simulink model "EXP7_Part2"  (R2018a)
settings: Solver=VariableStepAuto  StartTime=0.0  StopTime=0.2  RelTol=1e-3
undefined symbols (not defined in the file): DiscIntNeverNeededParam
libraries: dsparch4 x1, commsynccomp2 x1, dspsrcs4 x1
settings Model: Creator=user  LastModifiedBy=shohan

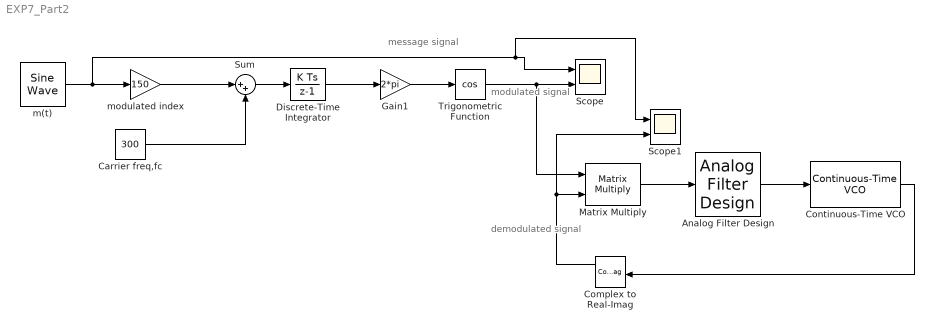
== system EXP7_Part2 ==
  note: modulated signal
  note: message signal
  note: demodulated
      | signal
  Analog Filter Design : dsparch4/Analog Filter Design  method=Butterworth  filttype=Lowpass  N=10  Wlo=2*pi*5  Whi=80  Rp=2  Rs=40
  Carrier freq,fc : Constant  Value=300
  Complex to Real-Imag : ComplexToRealImag
  Continuous-Time VCO : commsynccomp2/Continuous-Time VCO  Ac=1  Fc=10  Kc=50  Ph=0
      settings: SourceProductName=Communications System Toolbox  SourceProductBaseCode=CM
  Discrete-Time Integrator : DiscreteIntegrator  SampleTime=1/98000  ICPrevOutput=DiscIntNeverNeededParam  ICPrevScaledInput=DiscIntNeverNeededParam
  Gain1 : Gain  Gain=2*pi
  Matrix Multiply : Product  Multiplication=Matrix(*)
  Scope : Scope  NumInputPorts=2
  Scope1 : Scope  NumInputPorts=2
  Sum : Sum  Inputs=|++
  Trigonometric Function : Trigonometry  Operator=cos
  m(t) : dspsrcs4/Sine Wave  Amplitude=2  Frequency=10  Phase=pi/3  SampleMode=Discrete  OutComplex=Real  CompMethod=Trigonometric fcn  TableSize=Speed  SampleTime=1/98000  SamplesPerFrame=1  ResetState=Restart at time zero  OutputFrames=off  dataType=double  wordLen=16  udDataType=sfix(16)  fracBitsMode=Best precision  numFracBits=15  OutDataTypeStr=double  LastOutDataTypeStr=double
  modulated index : Gain  Gain=150
  wires:
  m(t)/1 -> Scope1/1, Scope/1, modulated index/1
  modulated index/1 -> Sum/1
  Carrier freq,fc/1 -> Sum/2
  Sum/1 -> Discrete-Time Integrator/1
  Discrete-Time Integrator/1 -> Gain1/1
  Gain1/1 -> Trigonometric Function/1
  Trigonometric Function/1 -> Matrix Multiply/1, Scope/2
  Matrix Multiply/1 -> Analog Filter Design/1
  Analog Filter Design/1 -> Continuous-Time VCO/1
  Continuous-Time VCO/1 -> Complex to Real-Imag/1
  Complex to Real-Imag/1 -> Matrix Multiply/2, Scope1/2
